simulink model "Repetitive_01"  (Simulink 7.1)
settings: Solver=ode45  StartTime=0.0  StopTime=10.0  RelTol=1e-3
CloseFcn:
  | rtwprivate ssgencode ModelCloseRequest untitled
settings Model: Creator=Meisel  LastModifiedBy=Meisel

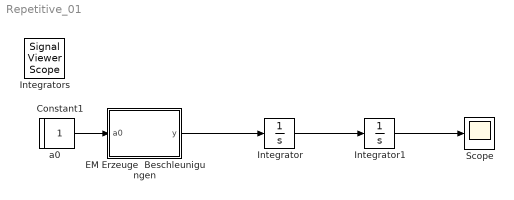
== system Repetitive_01 ==
  EM Erzeuge  Beschleunigungen : Stateflow chart
  Integrator : Integrator
  Integrator1 : Integrator
  Scope : Scope
      settings: TimeRange=10  YMin=0  YMax=60
  a0 : Constant  Value=0.1  OutDataType=sfix(16)  OutScaling=2^0
  Constant1 : Constant  IOType=siggen  OutDataType=sfix(16)  OutScaling=2^0
  Integrators : SignalViewerScope  IOType=viewer  NumInputPorts=2  RefreshTime=0.035000
      settings: TimeRange=10  YMin=0~0  YMax=10~60
  wires:
  EM Erzeuge  Beschleunigungen/1(y) -> Integrator/1
  Integrator/1 -> Integrator1/1
  Integrator1/1 -> Scope/1
  a0/1 -> EM Erzeuge  Beschleunigungen/1(a0)

== matlab function EM Erzeuge Beschleunigungen ==
  data: y output double; a0 input double
function y = fcn(a0)
% Embedded MATLAB block

k=10;          % muss konstant sein
m=zeros(1,k);  % m erzeugen

% Massen Initialisieren
for i=1:k
    m(i) = i*a0;
end

y = m;
